simulink library "Pressure_Drop_StoragePipe"  (Simulink 8.2)
settings: Solver=ode45  StartTime=0.0  StopTime=10.0  RelTol=1e-3
undefined symbols (not defined in the file): dia, hgt
libraries: carnot x2
settings Model: Creator=drhf  LastModifiedBy=drhf

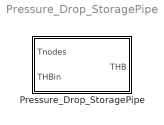
== system Pressure_Drop_StoragePipe ==
  Pressure_Drop_StoragePipe : Subsystem  mask(Pressure drop pipe connection of a storage){dia=dia, hgt=hgt}
      mask prompts: dia "Diameter in m"; hgt "height difference inlet-outlet"
      mask help:
      | Calculates the pressure drop in a pipe connection to a storage according to:
      | dp = qua*mdot^2 + lin*mdot + density*grav*height
      | The temperature for the density is taken from the storage nodes.
      mask Help: web(fullfile(path_carnot('help'),'Pressure_Drop_StoragePipe.html'),'-helpbrowser')

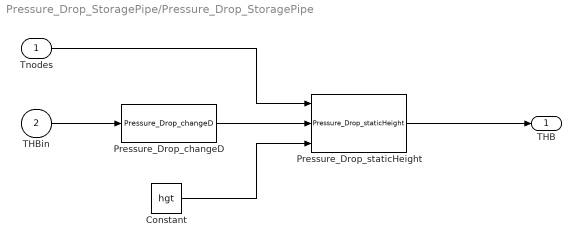
== system Pressure_Drop_StoragePipe/Pressure_Drop_StoragePipe ==
  Tnodes : Inport
  THBin : Inport  Port=2
  Constant : Constant  Value=hgt
  Pressure_Drop_changeD : carnot/Basic/Pressure_Drop/Pressure_Drop_changeD  dia=dia
  Pressure_Drop_staticHeight : carnot/Basic/Pressure_Drop/Pressure_Drop_staticHeight
  THB : Outport
  wires:
  Pressure_Drop_staticHeight/1 -> THB/1
  Tnodes/1 -> Pressure_Drop_staticHeight/1
  Pressure_Drop_changeD/1 -> Pressure_Drop_staticHeight/2
  Constant/1 -> Pressure_Drop_staticHeight/3
  THBin/1 -> Pressure_Drop_changeD/1
